simulink model "GCU_Model_genCode"  (R2018a)
settings: Solver=FixedStepDiscrete  StartTime=0.0  StopTime=20  FixedStep=0.0002  RelTol=1e-3  EnableMultiTasking=on
libraries: simulink x3, uartLib x2, clutchMotorLib x1, efiLib x1, engineControlLib x1, gearMotorLib x1
(part 1 of 2)
settings Model: Creator=SIMONE  LastModifiedBy=SIMONE
settings SolverCC: AutoInsertRateTranBlk=on
settings OptimizationCC: DefaultParameterBehavior=Inlined  UseDivisionForNetSlopeComputation=on  UseFloatMulNetSlope=on  InlineInvariantSignals=on  PassReuseOutputArgsAs=Individual arguments  ZeroExternalMemoryAtStartup=off  ZeroInternalMemoryAtStartup=off  NoFixptDivByZeroProtection=on  EfficientFloat2IntCast=on  LifeSpan=1  OptimizeBlockOrder=speed  DifferentSizesBufferReuse=on
settings DebuggingCC: ParameterTunabilityLossMsg=error
settings HardwareCC: ProdBitPerPointer=32  ProdBitPerSizeT=32  ProdBitPerPtrDiffT=32  ProdLargestAtomicInteger=Long  ProdLargestAtomicFloat=Double  ProdWordSize=32  ProdLongLongMode=on  ProdHWDeviceType=ARM Compatible->ARM Cortex
settings SFSimCC: MATLABDynamicMemAlloc=off
settings RTWCC: SystemTargetFile=ert.tlc  TemplateMakefile=ert_default_tmf  GenerateReport=on  IncludeHyperlinkInReport=on  LaunchReport=on  GenerateTraceInfo=on  GenerateTraceReport=on  GenerateTraceReportSl=on  GenerateTraceReportSf=on  GenerateTraceReportEml=on  GenerateCodeMetricsReport=on
settings CodeAppCC: ForceParamTrailComments=on  IgnoreCustomStorageClasses=off  OperatorAnnotations=on  SimulinkDataObjDesc=on  SFDataObjDesc=on  CustomSymbolStrGlobalVar=rt$N$M  CustomSymbolStrType=$N$M  CustomSymbolStrFcn=$N$M$F  CustomSymbolStrMacro=$N$M  InsertBlockDesc=on
settings ERTTargetCC: TargetLangStandard=C99 (ISO)  GenerateSampleERTMain=on  IncludeMdlTerminateFcn=off  CombineSignalStateStructs=on  SupportAbsoluteTime=off  SupportComplex=off  SupportNonInlinedSFcns=on  InlinedParameterPlacement=NonHierarchical  ERTCustomFileTemplate=example_file_process.tlc  ERTFilePackagingFormat=CompactWithDataFile  MemSecPackage=Simulink

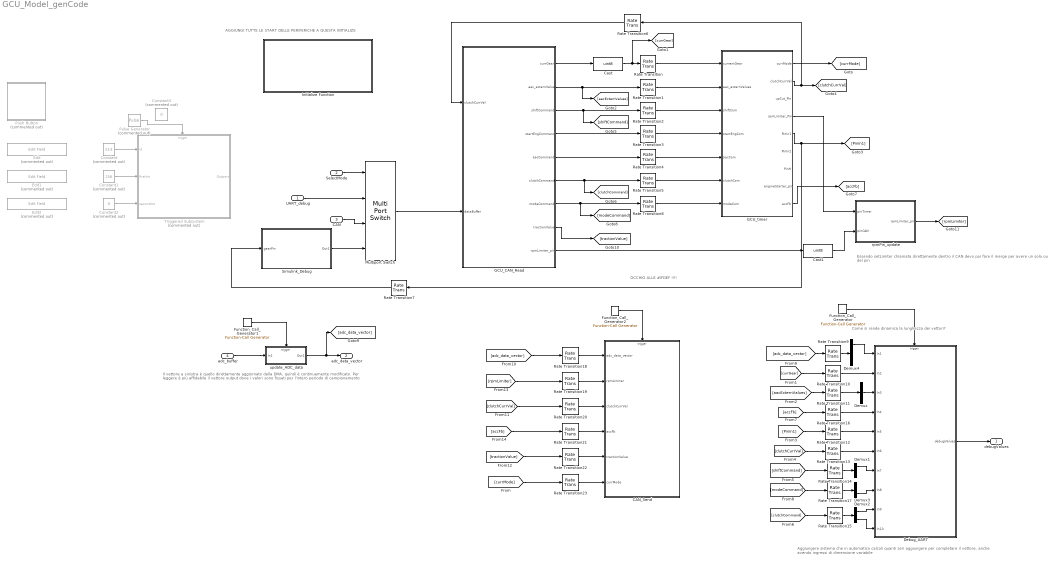
== system GCU_Model_genCode ==
  note: AGGIUNGI TUTTE LE START DELLE PERIFERICHE A QUESTA INITIALIZE
  note: Il vettore a sinistra è quello direttamente aggiornato dalla DMA, quindi è continuamente modificato.
      | Per leggere è più affidabile il vettore output dove i valori sono fissati per l'intero periodo di campionamento
  note: Come si rende dinamica la lunghezza dei vettori?
  note: Essendo setLimiter chiamata direttamente dentro il CAN devo poi fare il merge
      | per avere un solo output del pin
  note: OCCHIO ALLE #IFDEF !!!!
  note: Aggiungere sistema che in automatico calcoli quanti zeri aggiungere
      | per completare il vettore, anche avendo ingressi di dimensione variabile
  UART_debug : Inport  OutDataTypeStr=uint8  PortDimensions=10
  SelectMode : Inport  Port=2
  CAN : Inport  Port=3  OutDataTypeStr=uint8  PortDimensions=10
  adc_buffer : Inport  Port=4  OutDataTypeStr=uint32
  CAN_Send : Subsystem  TreatAsAtomicUnit=on
  Cast : DataTypeConversion  OutDataTypeStr=uint8
  Cast1 : DataTypeConversion  OutDataTypeStr=uint8
  Constant : Constant  Commented=on  Value=513  OutDataTypeStr=uint16
  Constant1 : Constant  Commented=on  Value=256  OutDataTypeStr=uint16
  Constant2 : Constant  Commented=on  Value=0  OutDataTypeStr=uint16
  Constant3 : Constant  Commented=on  Value=0
  "Debug_UART " : Subsystem  TreatAsAtomicUnit=on
  Demux : Demux  Outputs=3
  Demux1 : Demux  Outputs=2
  Demux2 : Demux  Outputs=2
  Demux3 : Demux  Outputs=2
  Demux4 : Demux  Outputs=10
  Edit : EditField  Commented=on  WebBlockId=879  LabelPosition=Hide  Alignment=Center
  Edit1 : EditField  Commented=on  WebBlockId=880  LabelPosition=Hide  Alignment=Center
  Edit2 : EditField  Commented=on  WebBlockId=881  LabelPosition=Hide  Alignment=Center
  Function_Call_Generator : simulink/Ports & Subsystems/Function-Call Generator  sample_time=[0.001, 0.0004]  numberOfIterations=1
  Function_Call_Generator1 : simulink/Ports & Subsystems/Function-Call Generator  sample_time=[0.001, 0.0006]  numberOfIterations=1
  Function_Call_Generator2 : simulink/Ports & Subsystems/Function-Call Generator  sample_time=[0.001, 0.0008]  numberOfIterations=1
  GCU_CAN_Read : Subsystem  TreatAsAtomicUnit=on  SystemSampleTime=[0.001, 0.0002]
  GCU_timer : Subsystem  TreatAsAtomicUnit=on  SystemSampleTime=0.001
  Initialize Function : Subsystem  TreatAsAtomicUnit=on
  Multiport Switch : MultiPortSwitch  DiagnosticForDefault=Warning
  Pulse Generator : DiscretePulseGenerator  Commented=on  PulseType=Time based  Period=1000  PulseWidth=0.1  PhaseDelay=1
  Push Button : Subsystem  Commented=on  DialogController=hmiCreateDDGDialog  IsWebBlock=on  mask(MWDashboardBlock){webBlockId=12b47424-de0c-4dac-be92-db9266863398, webBlockType=pushbutton, ShowInLibBrwoser=on, ShowInitialText=on, HMISrcModelName=GCU_Model_genCode}
      mask prompts: webBlockId "WebBlock Id"; webBlockType "WebBlock Type"; HMISrcModelName "Source Model"
      mask help: SimulinkHMI:dialogs:PushButtonDialogDesc
      mask Help: helpview([docroot '/mapfiles/simulink.map'], 'hmi_push_button')
      mask Display:
      | model = bdroot(gcb);
      | if strcmp(get_param(model,'BlockDiagramType'), 'library')
      |     image([(matlabroot) '/toolbox/simulink/hmi/icons/PushButton.png']);
      | end
  Rate Transition{,1..23} (24 alike) : RateTransition  Deterministic=off
  Simulink_Debug : Subsystem  TreatAsAtomicUnit=on  SystemSampleTime=[0.001, 0.0002]
  Triggered Subsystem : Subsystem  Commented=on  TreatAsAtomicUnit=on
  rpmPin_update : Subsystem
  update_ADC_data : Subsystem  TreatAsAtomicUnit=on
  "debugValues " : Outport
  adc_data_vector : Outport  Port=2  OutDataTypeStr=uint32
  wires:
  GCU_CAN_Read/9(rpmLimiter_pin) -> Cast1/1
  GCU_CAN_Read/4(startEngCommand) -> Rate Transition3/1
  Multiport Switch/1 -> GCU_CAN_Read/2(dataBuffer)
  Rate Transition8/1 -> GCU_timer/7(modeCom)
  Rate Transition/1 -> GCU_timer/1(currentGear)
  Cast/1 -> [currGear], Rate Transition/1
  GCU_CAN_Read/7(modeCommand) -> [modeCommand], Rate Transition8/1
  GCU_timer/5(PinIn1) -> Rate Transition7/1, [PinIn1]
  Rate Transition4/1 -> GCU_timer/5(aacCom)
  GCU_CAN_Read/2(aac_externValue) -> [aacExternValues], Rate Transition1/1
  GCU_CAN_Read/3(shiftCommand) -> [shiftCommand], Rate Transition2/1
  GCU_timer/2(clutchCurrVal) -> [clutchCurrVal], Rate Transition6/1
  Cast1/1 -> rpmPin_update/2(pinCAN)
  Rate Transition5/1 -> GCU_timer/6(clutchCom)
  GCU_CAN_Read/1(currGear) -> Cast/1
  Rate Transition2/1 -> GCU_timer/3(shiftCom)
  Rate Transition1/1 -> GCU_timer/2(aac_externValues)
  GCU_timer/4(rpmLimiter_Pin) -> rpmPin_update/1(pinTimer)
  GCU_CAN_Read/6(clutchCommand) -> [clutchCommand], Rate Transition5/1
  GCU_CAN_Read/5(aacCommand) -> Rate Transition4/1
  Rate Transition6/1 -> GCU_CAN_Read/1(clutchCurrVal)
  Rate Transition3/1 -> GCU_timer/4(startEngCom)
  Function_Call_Generator/1 -> "Debug_UART "/Trigger
  "Debug_UART "/1(debugValues) -> "debugValues "/1
  Rate Transition10/1 -> "Debug_UART "/2(In2)
  Rate Transition11/1 -> Demux/1
  Demux/2 -> "Debug_UART "/3(In3)
  Rate Transition7/1 -> Simulink_Debug/1(gearPin)
  Simulink_Debug/1(Out1) -> Multiport Switch/4
  GCU_timer/1(currMode) -> [currMode]
  [currGear] -> Rate Transition10/1
  [aacExternValues] -> Rate Transition11/1
  [PinIn1] -> Rate Transition12/1
  Rate Transition12/1 -> "Debug_UART "/5(In5)
  [clutchCurrVal] -> Rate Transition13/1
  Rate Transition13/1 -> "Debug_UART "/6(In6)
  [shiftCommand] -> Rate Transition14/1
  [clutchCommand] -> Rate Transition15/1
  Rate Transition14/1 -> Demux1/1
  Demux1/1 -> "Debug_UART "/7(In7)
  Demux2/1 -> "Debug_UART "/9(In9)
  Rate Transition15/1 -> Demux2/1
  Demux2/2 -> "Debug_UART "/10(In10)
  Constant/1 -> Triggered Subsystem/1(id)
  Constant2/1 -> Triggered Subsystem/3(secondInt)
  Constant1/1 -> Triggered Subsystem/2(firstInt)
  Pulse Generator/1 -> Triggered Subsystem/Trigger
  SelectMode/1 -> Multiport Switch/1
  UART_debug/1 -> Multiport Switch/2
  GCU_timer/9(accFb) -> [accFb]
  [accFb] -> Rate Transition16/1
  Rate Transition16/1 -> "Debug_UART "/4(In4)
  [modeCommand] -> Rate Transition17/1
  Rate Transition17/1 -> Demux3/1
  Demux3/2 -> "Debug_UART "/8(In8)
  CAN/1 -> Multiport Switch/3
  Function_Call_Generator1/1 -> update_ADC_data/Trigger
  adc_buffer/1 -> update_ADC_data/1(In1)
  update_ADC_data/1(Out1) -> [adc_data_vector], adc_data_vector/1
  [adc_data_vector] -> Rate Transition9/1
  Rate Transition9/1 -> Demux4/1
  Demux4/1 -> "Debug_UART "/1(In1)
  Function_Call_Generator2/1 -> CAN_Send/Trigger
  [adc_data_vector] -> Rate Transition18/1
  GCU_CAN_Read/8(tractionValue) -> [tractionValue]
  [currMode] -> Rate Transition23/1
  [clutchCurrVal] -> Rate Transition20/1
  [tractionValue] -> Rate Transition22/1
  rpmPin_update/1(rpmLimiter_pin) -> [rpmLimiter]
  [rpmLimiter] -> Rate Transition19/1
  [accFb] -> Rate Transition21/1
  Rate Transition18/1 -> CAN_Send/1(adc_data_vector)
  Rate Transition19/1 -> CAN_Send/2(rpmLimiter)
  Rate Transition20/1 -> CAN_Send/3(clutchCurrVal)
  Rate Transition21/1 -> CAN_Send/4(accFb)
  Rate Transition22/1 -> CAN_Send/5(tractionValue)
  Rate Transition23/1 -> CAN_Send/6(currMode)

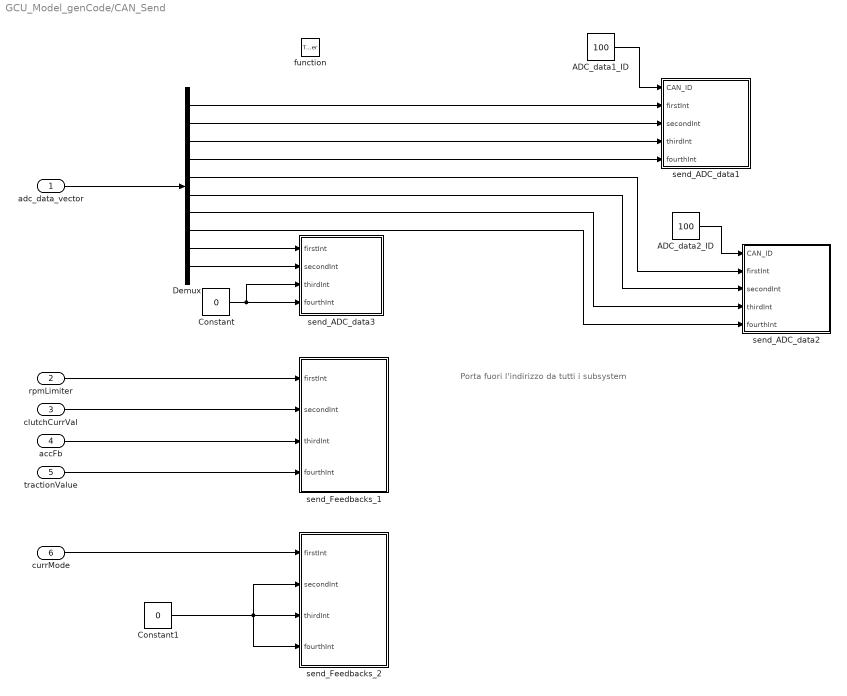
== system GCU_Model_genCode/CAN_Send ==
  note: Porta fuori l'indirizzo da tutti i subsystem
  adc_data_vector : Inport
  rpmLimiter : Inport  Port=2
  clutchCurrVal : Inport  Port=3
  accFb : Inport  Port=4
  tractionValue : Inport  Port=5
  currMode : Inport  Port=6
  function : TriggerPort  TriggerType=function-call  VariantControl=Variant
  ADC_data1_ID : Constant  Value=100  OutDataTypeStr=uint16
  ADC_data2_ID : Constant  Value=100  OutDataTypeStr=uint16
  Constant : Constant  Value=0  OutDataTypeStr=uint16
  Constant1 : Constant  Value=0  OutDataTypeStr=uint16
  Demux : Demux  Outputs=10
  send_ADC_data1 : Subsystem
  send_ADC_data2 : Subsystem
  send_ADC_data3 : Subsystem
  send_Feedbacks_1 : Subsystem
  send_Feedbacks_2 : Subsystem
  wires:
  adc_data_vector/1 -> Demux/1
  Demux/1 -> send_ADC_data1/2(firstInt)
  Demux/2 -> send_ADC_data1/3(secondInt)
  Demux/3 -> send_ADC_data1/4(thirdInt)
  Demux/4 -> send_ADC_data1/5(fourthInt)
  Demux/5 -> send_ADC_data2/2(firstInt)
  Demux/6 -> send_ADC_data2/3(secondInt)
  Demux/7 -> send_ADC_data2/4(thirdInt)
  Demux/8 -> send_ADC_data2/5(fourthInt)
  Demux/9 -> send_ADC_data3/1(firstInt)
  Demux/10 -> send_ADC_data3/2(secondInt)
  Constant/1 -> send_ADC_data3/3(thirdInt), send_ADC_data3/4(fourthInt)
  rpmLimiter/1 -> send_Feedbacks_1/1(firstInt)
  clutchCurrVal/1 -> send_Feedbacks_1/2(secondInt)
  accFb/1 -> send_Feedbacks_1/3(thirdInt)
  tractionValue/1 -> send_Feedbacks_1/4(fourthInt)
  currMode/1 -> send_Feedbacks_2/1(firstInt)
  Constant1/1 -> send_Feedbacks_2/4(fourthInt), send_Feedbacks_2/2(secondInt), send_Feedbacks_2/3(thirdInt)
  ADC_data1_ID/1 -> send_ADC_data1/1(CAN_ID)
  ADC_data2_ID/1 -> send_ADC_data2/1(CAN_ID)

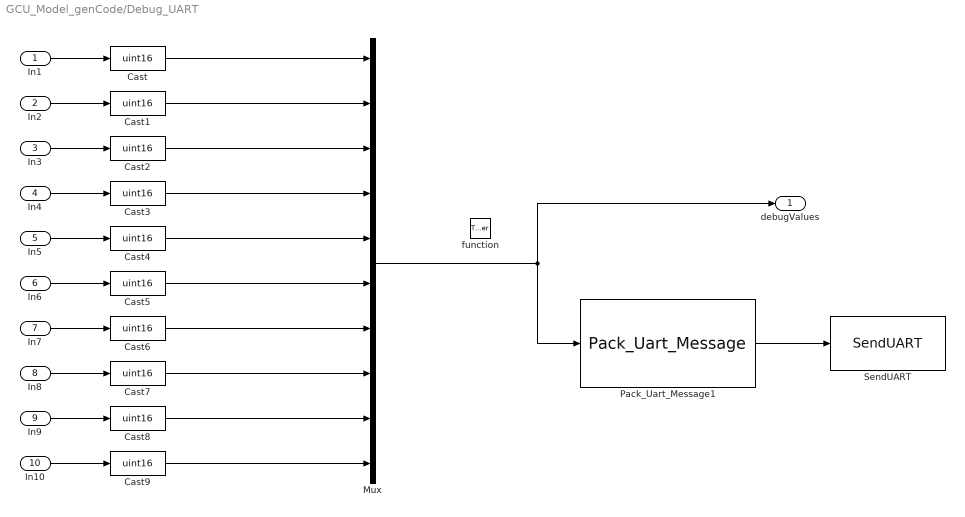
== system GCU_Model_genCode/Debug_UART  ==
  In1 : Inport
  In2 : Inport  Port=2
  In3 : Inport  Port=3
  In4 : Inport  Port=4
  In5 : Inport  Port=5
  In6 : Inport  Port=6
  In7 : Inport  Port=7
  In8 : Inport  Port=8
  In9 : Inport  Port=9
  In10 : Inport  Port=10
  function : TriggerPort  TriggerType=function-call  VariantControl=Variant
  Cast{,1..9} (10 alike) : DataTypeConversion  OutDataTypeStr=uint16
  Mux : Mux  Inputs=10
  Pack_Uart_Message1 : uartLib/Pack_Uart_Message  SFunctionModules=''
      settings: SourceProductName=GCU Library
  SendUART : uartLib/SendUART  SFunctionModules=''
      settings: SourceProductName=GCU Library
  debugValues : Outport
  wires:
  Pack_Uart_Message1/1 -> SendUART/1
  Mux/1 -> debugValues/1, Pack_Uart_Message1/1
  In1/1 -> Cast/1
  Cast/1 -> Mux/1
  In2/1 -> Cast1/1
  Cast1/1 -> Mux/2
  In3/1 -> Cast2/1
  Cast2/1 -> Mux/3
  Cast3/1 -> Mux/4
  In4/1 -> Cast3/1
  Cast4/1 -> Mux/5
  In5/1 -> Cast4/1
  Cast5/1 -> Mux/6
  In6/1 -> Cast5/1
  Cast6/1 -> Mux/7
  In7/1 -> Cast6/1
  Cast7/1 -> Mux/8
  In8/1 -> Cast7/1
  Cast8/1 -> Mux/9
  In9/1 -> Cast8/1
  Cast9/1 -> Mux/10
  In10/1 -> Cast9/1

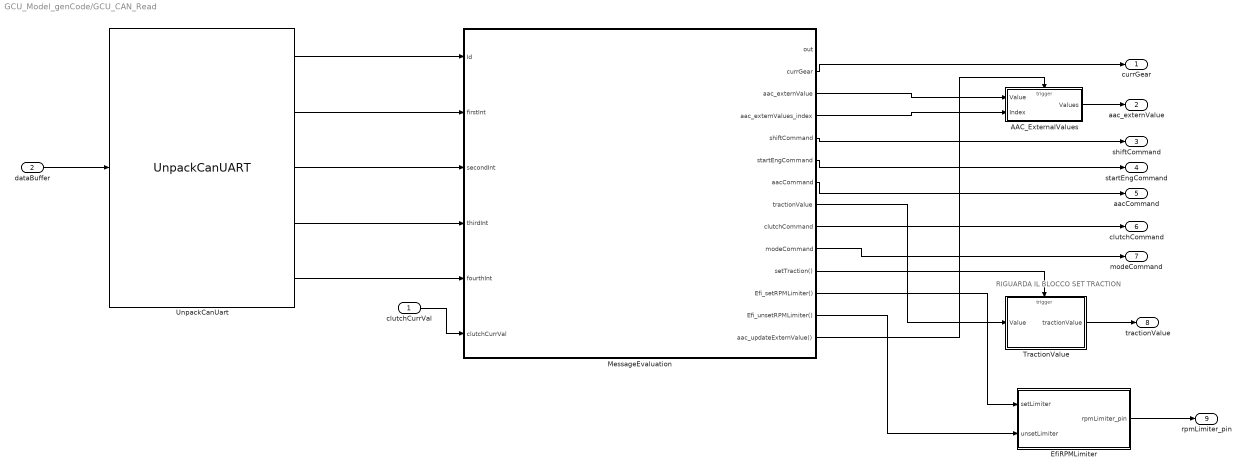
== system GCU_Model_genCode/GCU_CAN_Read ==
  note: RIGUARDA IL BLOCCO SET TRACTION
  clutchCurrVal : Inport
  dataBuffer : Inport  Port=2
  AAC_ExternalValues : Subsystem  TreatAsAtomicUnit=on
  EfiRPMLimiter : Subsystem
  MessageEvaluation : Stateflow chart  TreatAsAtomicUnit=on  SystemSampleTime=[0.001, 0.0002]
  TractionValue : Subsystem  TreatAsAtomicUnit=on
  UnpackCanUart : S-Function  FunctionName=UnpackCanUART  SFunctionDeploymentMode=off  EnableBusSupport=off
  currGear : Outport
  aac_externValue : Outport  Port=2
  shiftCommand : Outport  Port=3
  startEngCommand : Outport  Port=4
  aacCommand : Outport  Port=5
  clutchCommand : Outport  Port=6
  modeCommand : Outport  Port=7
  tractionValue : Outport  Port=8
  rpmLimiter_pin : Outport  Port=9
  wires:
  MessageEvaluation/12(Efi_setRPMLimiter()) -> EfiRPMLimiter/1(setLimiter)
  UnpackCanUart/4 -> MessageEvaluation/4(thirdInt)
  MessageEvaluation/4(aac_externValues_index) -> AAC_ExternalValues/2(Index)
  MessageEvaluation/13(Efi_unsetRPMLimiter()) -> EfiRPMLimiter/2(unsetLimiter)
  MessageEvaluation/7(aacCommand) -> aacCommand/1
  MessageEvaluation/9(clutchCommand) -> clutchCommand/1
  dataBuffer/1 -> UnpackCanUart/1
  MessageEvaluation/10(modeCommand) -> modeCommand/1
  MessageEvaluation/11(setTraction()) -> TractionValue/Trigger
  MessageEvaluation/5(shiftCommand) -> shiftCommand/1
  MessageEvaluation/3(aac_externValue) -> AAC_ExternalValues/1(Value)
  MessageEvaluation/8(tractionValue) -> TractionValue/1(Value)
  MessageEvaluation/6(startEngCommand) -> startEngCommand/1
  UnpackCanUart/1 -> MessageEvaluation/1(Id)
  UnpackCanUart/5 -> MessageEvaluation/5(fourthInt)
  TractionValue/1(tractionValue) -> tractionValue/1
  UnpackCanUart/3 -> MessageEvaluation/3(secondInt)
  clutchCurrVal/1 -> MessageEvaluation/6(clutchCurrVal)
  MessageEvaluation/2(currGear) -> currGear/1
  MessageEvaluation/14(aac_updateExternValue()) -> AAC_ExternalValues/Trigger
  UnpackCanUart/2 -> MessageEvaluation/2(firstInt)
  EfiRPMLimiter/1(rpmLimiter_pin) -> rpmLimiter_pin/1
  AAC_ExternalValues/1(Values) -> aac_externValue/1

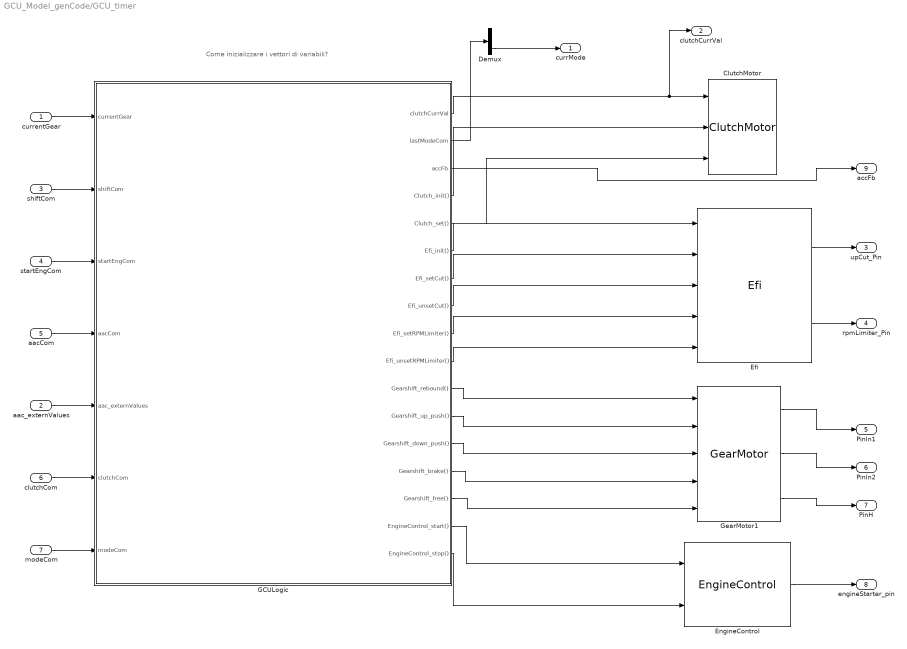
== system GCU_Model_genCode/GCU_timer ==
  note: Come inizializzare i vettori di variabili?
  currentGear : Inport
  aac_externValues : Inport  Port=2
  shiftCom : Inport  Port=3
  startEngCom : Inport  Port=4
  aacCom : Inport  Port=5
  clutchCom : Inport  Port=6
  modeCom : Inport  Port=7
  ClutchMotor : clutchMotorLib/ClutchMotor  SystemSampleTime=-1
      settings: SourceProductName=GCU Library
  Demux : Demux  Outputs=2
  Efi : efiLib/Efi
      settings: SourceProductName=GCU Library
  EngineControl : engineControlLib/EngineControl
      settings: SourceProductName=GCU Library
  GCULogic : Stateflow chart  TreatAsAtomicUnit=on
  GearMotor1 : gearMotorLib/GearMotor
      settings: SourceProductName=GCU Library
  currMode : Outport
  clutchCurrVal : Outport  Port=2
  upCut_Pin : Outport  Port=3
  rpmLimiter_Pin : Outport  Port=4
  PinIn1 : Outport  Port=5
  PinIn2 : Outport  Port=6
  PinH : Outport  Port=7
  engineStarter_pin : Outport  Port=8
  accFb : Outport  Port=9
  wires:
  GCULogic/17(EngineControl_stop()) -> EngineControl/2
  startEngCom/1 -> GCULogic/3(startEngCom)
  GCULogic/9(Efi_setRPMLimiter()) -> Efi/4
  GCULogic/6(Efi_init()) -> Efi/1
  clutchCom/1 -> GCULogic/6(clutchCom)
  GCULogic/16(EngineControl_start()) -> EngineControl/1
  GearMotor1/3 -> PinH/1
  GCULogic/10(Efi_unsetRPMLimiter()) -> Efi/5
  EngineControl/1 -> engineStarter_pin/1
  GCULogic/15(Gearshift_free()) -> GearMotor1/5
  GCULogic/14(Gearshift_brake()) -> GearMotor1/4
  GCULogic/11(Gearshift_rebound()) -> GearMotor1/1
  GearMotor1/2 -> PinIn2/1
  GearMotor1/1 -> PinIn1/1
  GCULogic/12(Gearshift_up_push()) -> GearMotor1/2
  shiftCom/1 -> GCULogic/2(shiftCom)
  aacCom/1 -> GCULogic/4(aacCom)
  GCULogic/4(Clutch_init()) -> ClutchMotor/2
  Efi/2 -> rpmLimiter_Pin/1
  GCULogic/7(Efi_setCut()) -> Efi/2
  Efi/1 -> upCut_Pin/1
  currentGear/1 -> GCULogic/1(currentGear)
  GCULogic/1(clutchCurrVal) -> ClutchMotor/1, clutchCurrVal/1
  GCULogic/8(Efi_unsetCut()) -> Efi/3
  GCULogic/5(Clutch_set()) -> ClutchMotor/3
  modeCom/1 -> GCULogic/7(modeCom)
  aac_externValues/1 -> GCULogic/5(aac_externValues)
  GCULogic/13(Gearshift_down_push()) -> GearMotor1/3
  GCULogic/3(accFb) -> accFb/1
  GCULogic/2(lastModeCom) -> Demux/1
  Demux/2 -> currMode/1

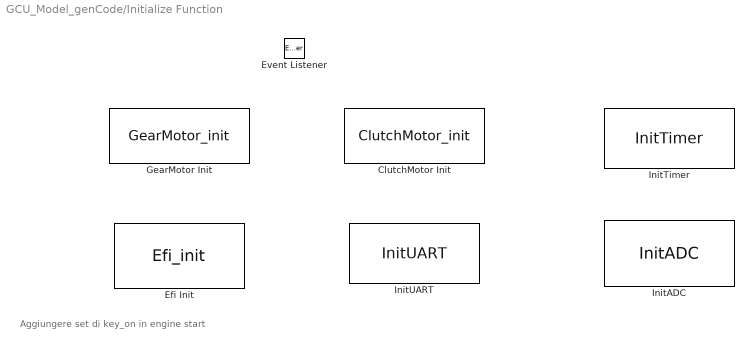
== system GCU_Model_genCode/Initialize Function ==
  note: Aggiungere set di key_on in engine start
  ClutchMotor Init : S-Function  FunctionName=ClutchMotor_init  SFunctionDeploymentMode=off  EnableBusSupport=off
  Efi Init : S-Function  FunctionName=Efi_init  SFunctionDeploymentMode=off  EnableBusSupport=off
  Event Listener : EventListener  DisableCoverage=on  EventName=reset
  GearMotor Init : S-Function  FunctionName=GearMotor_init  SFunctionDeploymentMode=off  EnableBusSupport=off
  InitADC : S-Function  FunctionName=InitADC  SFunctionDeploymentMode=off  EnableBusSupport=off
  InitTimer : S-Function  FunctionName=InitTimer  SFunctionDeploymentMode=off  EnableBusSupport=off
  InitUART : S-Function  FunctionName=InitUART  SFunctionDeploymentMode=off  EnableBusSupport=off

== system GCU_Model_genCode/Push Button ==

== system GCU_Model_genCode/Simulink_Debug ==
  gearPin : Inport
  AccelerationRoutine : Stateflow chart  TreatAsAtomicUnit=on  SystemSampleTime=[0.001, 0.0002]
  PackCanUart : S-Function  FunctionName=PackCanUART  SFunctionDeploymentMode=off  EnableBusSupport=off
  Out1 : Outport
  wires:
  PackCanUart/1 -> Out1/1
  AccelerationRoutine/2(firstInt) -> PackCanUart/2
  AccelerationRoutine/1(id) -> PackCanUart/1
  AccelerationRoutine/3(secondInt) -> PackCanUart/3
  gearPin/1 -> AccelerationRoutine/1(gearPin)

== system GCU_Model_genCode/Triggered Subsystem ==
  id : Inport
  firstInt : Inport  Port=2
  secondInt : Inport  Port=3
  Trigger : TriggerPort  VariantControl=Variant
  PackCanUart : S-Function  FunctionName=PackCanUART  SFunctionDeploymentMode=off  EnableBusSupport=off
  Scope : Scope
  Outport : Outport
  wires:
  PackCanUart/1 -> Outport/1, Scope/1
  id/1 -> PackCanUart/1
  firstInt/1 -> PackCanUart/2
  secondInt/1 -> PackCanUart/3

== system GCU_Model_genCode/rpmPin_update ==
  pinTimer : Inport
  pinCAN : Inport  Port=2
  Merge : Merge
  Rate Transition : RateTransition  Deterministic=off
  Triggered_Subsystem : Subsystem  TreatAsAtomicUnit=on
  Triggered_Subsystem1 : Subsystem  TreatAsAtomicUnit=on
  rpmLimiter_pin : Outport
  wires:
  pinTimer/1 -> Triggered_Subsystem/1(In1), Triggered_Subsystem/Trigger
  pinCAN/1 -> Rate Transition/1
  Triggered_Subsystem/1(Out1) -> Merge/1
  Triggered_Subsystem1/1(Out1) -> Merge/2
  Merge/1 -> rpmLimiter_pin/1
  Rate Transition/1 -> Triggered_Subsystem1/1(In1), Triggered_Subsystem1/Trigger

== system GCU_Model_genCode/update_ADC_data ==
  In1 : Inport
  function : TriggerPort  TriggerType=function-call  VariantControl=Variant
  update_ADC_data : S-Function  FunctionName=update_ADC_data  SFunctionDeploymentMode=off  EnableBusSupport=off
  Out1 : Outport
  wires:
  In1/1 -> update_ADC_data/1
  update_ADC_data/1 -> Out1/1

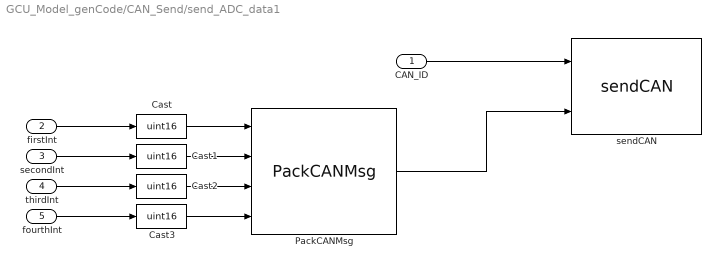
== system GCU_Model_genCode/CAN_Send/send_ADC_data1 ==
  CAN_ID : Inport
  firstInt : Inport  Port=2
  secondInt : Inport  Port=3
  thirdInt : Inport  Port=4
  fourthInt : Inport  Port=5
  Cast{,1..3} (4 alike) : DataTypeConversion  OutDataTypeStr=uint16
  PackCANMsg : S-Function  FunctionName=PackCANMsg  SFunctionDeploymentMode=off  EnableBusSupport=off
  sendCAN : S-Function  FunctionName=sendCAN  SFunctionDeploymentMode=off  EnableBusSupport=off
  wires:
  CAN_ID/1 -> sendCAN/1
  PackCANMsg/1 -> sendCAN/2
  firstInt/1 -> Cast/1
  secondInt/1 -> Cast1/1
  thirdInt/1 -> Cast2/1
  fourthInt/1 -> Cast3/1
  Cast/1 -> PackCANMsg/1
  Cast1/1 -> PackCANMsg/2
  Cast2/1 -> PackCANMsg/3
  Cast3/1 -> PackCANMsg/4

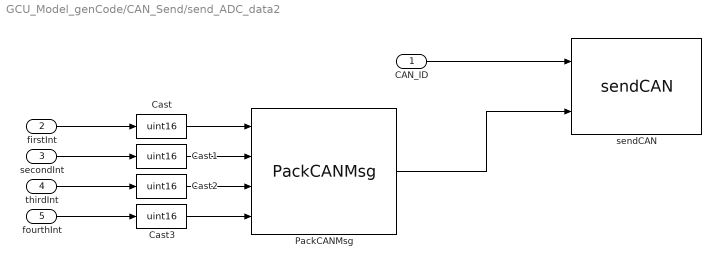
== system GCU_Model_genCode/CAN_Send/send_ADC_data2 ==
  CAN_ID : Inport
  firstInt : Inport  Port=2
  secondInt : Inport  Port=3
  thirdInt : Inport  Port=4
  fourthInt : Inport  Port=5
  Cast{,1..3} (4 alike) : DataTypeConversion  OutDataTypeStr=uint16
  PackCANMsg : S-Function  FunctionName=PackCANMsg  SFunctionDeploymentMode=off  EnableBusSupport=off
  sendCAN : S-Function  FunctionName=sendCAN  SFunctionDeploymentMode=off  EnableBusSupport=off
  wires:
  CAN_ID/1 -> sendCAN/1
  PackCANMsg/1 -> sendCAN/2
  firstInt/1 -> Cast/1
  secondInt/1 -> Cast1/1
  thirdInt/1 -> Cast2/1
  fourthInt/1 -> Cast3/1
  Cast/1 -> PackCANMsg/1
  Cast1/1 -> PackCANMsg/2
  Cast2/1 -> PackCANMsg/3
  Cast3/1 -> PackCANMsg/4

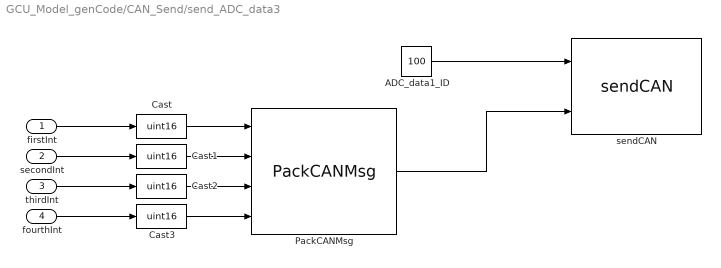
== system GCU_Model_genCode/CAN_Send/send_ADC_data3 ==
  firstInt : Inport
  secondInt : Inport  Port=2
  thirdInt : Inport  Port=3
  fourthInt : Inport  Port=4
  ADC_data1_ID : Constant  Value=100  OutDataTypeStr=uint16
  Cast{,1..3} (4 alike) : DataTypeConversion  OutDataTypeStr=uint16
  PackCANMsg : S-Function  FunctionName=PackCANMsg  SFunctionDeploymentMode=off  EnableBusSupport=off
  sendCAN : S-Function  FunctionName=sendCAN  SFunctionDeploymentMode=off  EnableBusSupport=off
  wires:
  ADC_data1_ID/1 -> sendCAN/1
  PackCANMsg/1 -> sendCAN/2
  firstInt/1 -> Cast/1
  secondInt/1 -> Cast1/1
  thirdInt/1 -> Cast2/1
  fourthInt/1 -> Cast3/1
  Cast/1 -> PackCANMsg/1
  Cast1/1 -> PackCANMsg/2
  Cast2/1 -> PackCANMsg/3
  Cast3/1 -> PackCANMsg/4

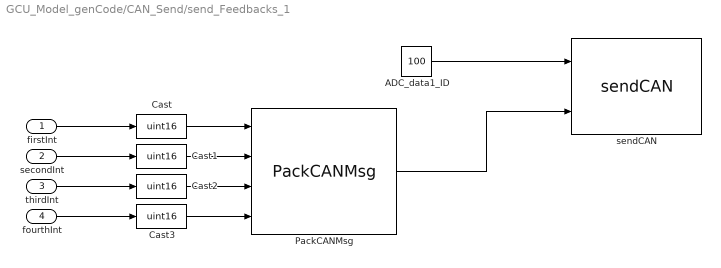
== system GCU_Model_genCode/CAN_Send/send_Feedbacks_1 ==
  firstInt : Inport
  secondInt : Inport  Port=2
  thirdInt : Inport  Port=3
  fourthInt : Inport  Port=4
  ADC_data1_ID : Constant  Value=100  OutDataTypeStr=uint16
  Cast{,1..3} (4 alike) : DataTypeConversion  OutDataTypeStr=uint16
  PackCANMsg : S-Function  FunctionName=PackCANMsg  SFunctionDeploymentMode=off  EnableBusSupport=off
  sendCAN : S-Function  FunctionName=sendCAN  SFunctionDeploymentMode=off  EnableBusSupport=off
  wires:
  ADC_data1_ID/1 -> sendCAN/1
  PackCANMsg/1 -> sendCAN/2
  firstInt/1 -> Cast/1
  secondInt/1 -> Cast1/1
  thirdInt/1 -> Cast2/1
  fourthInt/1 -> Cast3/1
  Cast/1 -> PackCANMsg/1
  Cast1/1 -> PackCANMsg/2
  Cast2/1 -> PackCANMsg/3
  Cast3/1 -> PackCANMsg/4

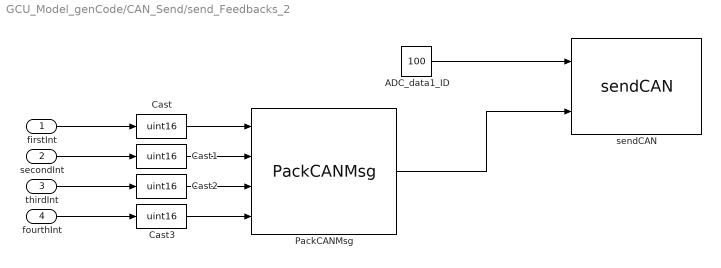
== system GCU_Model_genCode/CAN_Send/send_Feedbacks_2 ==
  firstInt : Inport
  secondInt : Inport  Port=2
  thirdInt : Inport  Port=3
  fourthInt : Inport  Port=4
  ADC_data1_ID : Constant  Value=100  OutDataTypeStr=uint16
  Cast{,1..3} (4 alike) : DataTypeConversion  OutDataTypeStr=uint16
  PackCANMsg : S-Function  FunctionName=PackCANMsg  SFunctionDeploymentMode=off  EnableBusSupport=off
  sendCAN : S-Function  FunctionName=sendCAN  SFunctionDeploymentMode=off  EnableBusSupport=off
  wires:
  ADC_data1_ID/1 -> sendCAN/1
  PackCANMsg/1 -> sendCAN/2
  firstInt/1 -> Cast/1
  secondInt/1 -> Cast1/1
  thirdInt/1 -> Cast2/1
  fourthInt/1 -> Cast3/1
  Cast/1 -> PackCANMsg/1
  Cast1/1 -> PackCANMsg/2
  Cast2/1 -> PackCANMsg/3
  Cast3/1 -> PackCANMsg/4

== system GCU_Model_genCode/GCU_CAN_Read/AAC_ExternalValues ==
  Value : Inport
  Index : Inport  Port=2
  function : TriggerPort  TriggerType=function-call  VariantControl=Variant
  Assignment : Assignment  IndexMode=Zero-based  DiagnosticForDimensions=Warning  IndexOptions=Index vector (port)  Indices=1  OutputSizes=1
  Unit Delay : UnitDelay  InitialCondition=[0,0,0]  SampleTime=-1
  Values : Outport
  wires:
  Assignment/1 -> Unit Delay/1, Values/1
  Unit Delay/1 -> Assignment/1
  Value/1 -> Assignment/2
  Index/1 -> Assignment/3

== system GCU_Model_genCode/GCU_CAN_Read/EfiRPMLimiter ==
  setLimiter : Inport
  unsetLimiter : Inport  Port=2
  Efi_setRpmLimiter : Subsystem  TreatAsAtomicUnit=on
  Efi_unsetRpmLimiter : Subsystem  TreatAsAtomicUnit=on
  Merge : Merge
  rpmLimiter_pin : Outport
  wires:
  setLimiter/1 -> Efi_setRpmLimiter/Trigger
  unsetLimiter/1 -> Efi_unsetRpmLimiter/Trigger
  Efi_unsetRpmLimiter/1(rpmLimiter_pin) -> Merge/2
  Efi_setRpmLimiter/1(rpmLimiter_pin) -> Merge/1
  Merge/1 -> rpmLimiter_pin/1

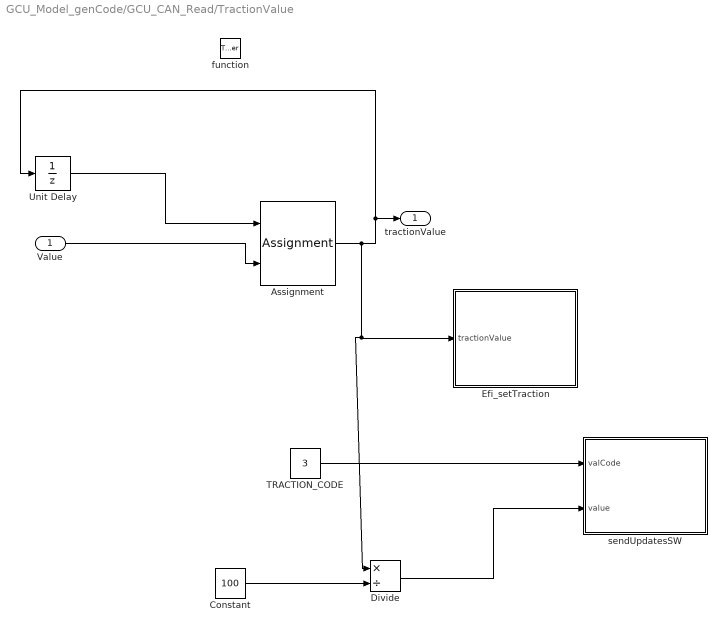
== system GCU_Model_genCode/GCU_CAN_Read/TractionValue ==
  Value : Inport
  function : TriggerPort  TriggerType=function-call  VariantControl=Variant
  Assignment : Assignment  IndexMode=Zero-based  DiagnosticForDimensions=Warning  IndexOptions=Index vector (dialog)  Indices=0  OutputSizes=1
  Constant : Constant  Value=100  OutDataTypeStr=uint16
  Divide : Product  Inputs=*/
  Efi_setTraction : Subsystem
  TRACTION_CODE : Constant  Value=3  OutDataTypeStr=uint16
  Unit Delay : UnitDelay  SampleTime=-1
  sendUpdatesSW : Subsystem
  tractionValue : Outport
  wires:
  Value/1 -> Assignment/2
  Assignment/1 -> Divide/1, Efi_setTraction/1(tractionValue), Unit Delay/1, tractionValue/1
  Unit Delay/1 -> Assignment/1
  TRACTION_CODE/1 -> sendUpdatesSW/1(valCode)
  Constant/1 -> Divide/2
  Divide/1 -> sendUpdatesSW/2(value)

== system GCU_Model_genCode/GCU_timer/GCULogic/sendUpdatesSW ==
  valCode : Inport  OutDataTypeStr=uint16  PortDimensions=1
  value : Inport  Port=2  OutDataTypeStr=uint16  PortDimensions=1
  f : TriggerPort  TriggerType=function-call  VariantControl=(inherit)
      settings: CopyFcn=Stateflow.SLINSF.SimulinkMan.removeBlockPreDeleteFcn  PreDeleteFcn=Stateflow.SLINSF.SimulinkMan.unsafePredeleteFcn
  GCU_FEEDBACK_ID : Constant  Value=793  OutDataTypeStr=uint16
  PackCanUart : S-Function  FunctionName=PackCanUART  SFunctionDeploymentMode=off  EnableBusSupport=off
  wires:
  GCU_FEEDBACK_ID/1 -> PackCanUart/1
  valCode/1 -> PackCanUart/2
  value/1 -> PackCanUart/3

== system GCU_Model_genCode/rpmPin_update/Triggered_Subsystem ==
  In1 : Inport
  Trigger : TriggerPort  TriggerType=either  VariantControl=Variant
  Out1 : Outport
  wires:
  In1/1 -> Out1/1

== system GCU_Model_genCode/rpmPin_update/Triggered_Subsystem1 ==
  In1 : Inport
  Trigger : TriggerPort  TriggerType=either  VariantControl=Variant
  Out1 : Outport
  wires:
  In1/1 -> Out1/1

== system GCU_Model_genCode/GCU_CAN_Read/EfiRPMLimiter/Efi_setRpmLimiter ==
  function : TriggerPort  TriggerType=function-call  VariantControl=Variant
  Efi SetRPMLimiter : S-Function  FunctionName=Efi_setRPMLimiter  SFunctionDeploymentMode=off  EnableBusSupport=off
  rpmLimiter_pin : Outport
  wires:
  Efi SetRPMLimiter/1 -> rpmLimiter_pin/1

== system GCU_Model_genCode/GCU_CAN_Read/EfiRPMLimiter/Efi_unsetRpmLimiter ==
  function : TriggerPort  TriggerType=function-call  VariantControl=Variant
  Efi UnSetRPMLimiter : S-Function  FunctionName=Efi_unsetRPMLimiter  SFunctionDeploymentMode=off  EnableBusSupport=off
  rpmLimiter_pin : Outport
  wires:
  Efi UnSetRPMLimiter/1 -> rpmLimiter_pin/1

== system GCU_Model_genCode/GCU_CAN_Read/TractionValue/Efi_setTraction ==
  tractionValue : Inport  OutDataTypeStr=uint16  PortDimensions=1
  GCU_TRACTION_CONTROL_EFI_ID : Constant  Value=1280  OutDataTypeStr=uint16
  PackCanUart : S-Function  FunctionName=PackCanUART  SFunctionDeploymentMode=off  EnableBusSupport=off
  wires:
  GCU_TRACTION_CONTROL_EFI_ID/1 -> PackCanUart/1
  tractionValue/1 -> PackCanUart/2

== system GCU_Model_genCode/GCU_CAN_Read/TractionValue/sendUpdatesSW ==
  valCode : Inport  OutDataTypeStr=uint16  PortDimensions=1
  value : Inport  Port=2  OutDataTypeStr=uint16  PortDimensions=1
  GCU_FEEDBACK_ID : Constant  Value=793  OutDataTypeStr=uint16
  PackCanUart : S-Function  FunctionName=PackCanUART  SFunctionDeploymentMode=off  EnableBusSupport=off
  wires:
  GCU_FEEDBACK_ID/1 -> PackCanUart/1
  value/1 -> PackCanUart/3
  valCode/1 -> PackCanUart/2

== stateflow chart GCU_Model_genCode/GCU_timer/GCULogic ==
  settings: updateMethod=DISCRETE  sampleTime=0.001
  state MODES [parallel]
    settings: executionOrder=1
    state MANUAL_MODES
      entry:
      lastModeCom[0] = modeCom[0];
      lastModeCom[1] = modeCom[1];
      entry, during:
      checkShift();
      checkClutch();
      state AUTOCROSS
      state ENDURANCE
      state SKIDPAD
      (default) -> ENDURANCE
    state INIT
    note: numeri delle modalità da decidere
    state checkClutch [function]
      (default) -> (junction 649)
      (junction 649) -> (junction 648) [order 1] : [clutchCom[0] ~= lastClutchCom]
      (junction 649) -> (junction 683) [order 2]
      (junction 648) -> (junction 682)
      (junction 682) -> (junction 687) [order 1] : [(~in(GEARSHIFT.DOWNSHIFTING) && ~in(NEUTRAL_STATE.SET_NEUTRAL)) || in(NEUTRAL_STATE.UNSET_NEUTRAL)]
      (junction 682) -> (junction 689) [order 2]
      (junction 687) -> (junction 691) : {lastClutchCom = clutchCom[0];
          |  Clutch_setValue(clutchCom[1]);}
    note: In caso di problema si riporta in endurance
    state checkShift [function]
      (default) -> (junction 635)
      (junction 635) -> (junction 637) [order 1] : [shiftCom[0] ~= lastShiftCom]
      (junction 635) -> (junction 641) [order 2]
      (junction 637) -> (junction 448) : {lastShiftCom = shiftCom[0];}
      (junction 448) -> (junction 450) [order 1] : [ shiftCom[1] == GEAR_COMMAND_UP]
      (junction 448) -> (junction 454) [order 2]
      (junction 450) -> (junction 452) : {send(GearshiftUp, NEUTRAL_STATE);
          |  send(GearshiftUp, GEARSHIFT);}
      (junction 454) -> (junction 456) [order 1] : [shiftCom[1] == GEAR_COMMAND_DOWN]
      (junction 454) -> (junction 460) [order 2]
      (junction 456) -> (junction 458) : {send(GearshiftDown, NEUTRAL_STATE);
          |  send(GearshiftDown, GEARSHIFT);}
      (junction 460) -> (junction 462) [order 1] : [shiftCom[1] == GEAR_COMMAND_NEUTRAL_UP]
      (junction 460) -> (junction 466) [order 2]
      (junction 462) -> (junction 464) : {send(GearshiftSetNeutral, NEUTRAL_STATE);
          |  send(GearshiftUp, GEARSHIFT);}
      (junction 466) -> (junction 469) [order 1] : [shiftCom[1] == GEAR_COMMAND_NEUTRAL_DOWN]
      (junction 466) -> (junction 473) [order 2]
      (junction 469) -> (junction 471) : {send(GearshiftSetNeutral, NEUTRAL_STATE);
          |  send(GearshiftDown, GEARSHIFT); }
    state ACCELERATION
      entry:
      lastModeCom[0] = modeCom[0];
      lastModeCom[1] = modeCom[1];
      state AAC
        note: Ricorda load dei default parameters
        note: Forse serve stato OFF, forse no
        note: ATTENZIONE: mancano delle istruzioni in alcuni stati
        note: E' giusto che clutch venga settata due volte?
        note: Riguarda funzionamento counter
        state ACTIVE
          note: Quindi continuo a settare Clutch?
          state START
            entry:
            accFb = 2;
            aacCounter = AAC_WORK_RATE_ms
            send(Efi_setRPMLimiter);
            Clutch_setValue(uint8(100));
            sendUpdatesSW(ACC_CODE, uint16(1));
            during:
            aacCounter = aacCounter - 1;
          state READY
            entry:
            accFb = 3;
            aacCounter = AAC_WORK_RATE_ms
            Clutch_setValue(uint8(100));
            during:
            aacCounter = aacCounter - 1;
            en, du:
            checkShift();
          note: SET blip è sbagliato
          state START_RELEASE
            entry:
            aac_clutchValue = double(getAacParam(RAMP_START));
            Clutch_setValue(uint8(aac_clutchValue));
            aac_dtRelease = getAacParam(RAMP_TIME) / int32(AAC_WORK_RATE_ms);
            aac_clutchStep = double((getAacParam(RAMP_START) - getAacParam(RAMP_END)) * int32(AAC_WORK_RATE_ms)) / double(getAacParam(RAMP_TIME));
            aacCounter = AAC_WORK_RATE_ms;
            sendUpdatesSW(ACC_CODE, uint16(2));
            during:
            aacCounter = aacCounter - 1;
          state RUNNING
            entry:
            aacCounter = AAC_WORK_RATE_ms
            lastShift =  currentGear;
            entry, during:
            aacCheckShift();
          note: Continuo a controllare ogni 25ms?
          state aacCheckShift [function]
            (default) -> (junction 716)
            (junction 716) -> (junction 717) [order 1] : [lastShift == currentGear]
            (junction 716) -> (junction 720) [order 2]
            (junction 717) -> (junction 593)
            (junction 593) -> (junction 604) [order 1] : [aac_externValues[int32(aac_values.RPM)] >= aac_parameters[ uint8(aac_params.RPM_LIMIT_1_2) + currentGear -1]]
            (junction 593) -> (junction 606) [order 2]
            (junction 604) -> (junction 608)
            (junction 608) -> (junction 610) [order 1] : [aac_externValues[int32(aac_values.WHEEL_SPEED)] >= aac_parameters[ uint8(aac_params.SPEED_LIMIT_1_2) + currentGear-1]]
            (junction 608) -> (junction 612) [order 2]
            (junction 610) -> (junction 614) : {send(GearshiftUp, GEARSHIFT); lastShift = lastShift + 1;}
          state RELEASING
            entry:
            aac_clutchValue = aac_clutchValue - aac_clutchStep;
            Clutch_setValue(uint8(aac_clutchValue));
            aac_dtRelease = aac_dtRelease - 1;
            aacCounter = AAC_WORK_RATE_ms;
            during:
            aacCounter = aacCounter - 1;
          note: Teniamo questa cosa di eseguire ogni 25ms? O calcoliamo direttamente
              | il Ttot?
          (default) -> MODES.ACCELERATION.AAC.ACTIVE.START
          (junction 558) -> READY [order 2]
          MODES.ACCELERATION.AAC.ACTIVE.START -> READY : [aacCounter <= 1]
          READY -> (junction 558) : [aacCounter <= 1]
          (junction 558) -> START_RELEASE [order 1] : [aacCom[0] ~= lastAacCom && aacCom[1] == RELEASE_AAC_COM]{lastAacCom = aacCom[0];}
          START_RELEASE -> RELEASING : [aacCounter <= 1]
          (junction 572) -> RUNNING [order 1] : [aac_dtRelease <= 0 || clutchCurrVal <= getAacParam(RAMP_END)]
              | {Clutch_setValue(uint8(0)); send(Efi_unsetRPMLimiter);}
          (junction 572) -> RELEASING [order 2]
          RELEASING -> (junction 572) : [aacCounter <=1]
        note: Quando devo fare clutch release?Forse risolto in CAN
        state STOPPING
          entry:
          send(Efi_unsetRPMLimiter);
          sendUpdatesSW(ACC_CODE, uint16(0));
        note: da verificare la marcia di uscita
        note: !!!!Gli array di MATLAB sono 1-based
        state param = getAacParam(index) [function]
          (default) -> (junction 566)
          (junction 566) -> (junction 570) : {param = aac_parameters[int32(index)]}
        ACTIVE -> STOPPING : [aacCom[0] ~= lastAacCom && aacCom[1] == STOP_AAC_COM]
            | {lastAacCom = aacCom[0]}
        RUNNING -> STOPPING : [currentGear == 5]
      state NotReady
        entry, during:
        accFb = 1;
        checkShift();
        checkClutch();
      note: prima di entrare svuotare il buffer
      (default) -> NotReady
      NotReady -> ACTIVE : [aacCom[0] ~= lastAacCom && aacCom[1] == START_AAC_COM]
          | {lastAacCom = aacCom[0]}
      STOPPING -> NotReady
    note: Stopping potrebbe essere esterno ad AAC,
        | Dove faccio unsetRPMLimiter?
    (junction 826) -> (junction 800)
    (default) -> MODES.INIT
    MODES.INIT -> (junction 800)
    (junction 800) -> AUTOCROSS [order 1] : [modeCom[1] == AUTOCROSS_MODE]
    (junction 800) -> (junction 808) [order 2]
    MANUAL_MODES -> (junction 826) : [modeCom[0] != lastModeCom[0] && modeCom[1] != lastModeCom[1]]
    ACCELERATION -> (junction 826) : [modeCom[0]~= lastModeCom[0] && modeCom[1] != lastModeCom[1]]
        | {send(Efi_unsetRPMLimiter)}
    (junction 808) -> ENDURANCE [order 1] : [modeCom[1] == ENDURANCE_MODE]
    (junction 808) -> (junction 812) [order 2]
    (junction 812) -> SKIDPAD [order 1] : [modeCom[1] == SKIDPAD_MODE]
    (junction 812) -> (junction 815) [order 2]
    (junction 815) -> MANUAL_MODES [order 2]
    (junction 815) -> ACCELERATION [order 1] : [modeCom[1] == ACC_MODE]
  note: DIVERSA DA QUELLA IN C E NON COMPLETA
  state sendUpdatesSW (valCode, value) [function]
  state NEUTRAL_STATE [parallel]
    settings: executionOrder=2
    state NEUTRAL
    state UNSET_NEUTRAL
    state SET_NEUTRAL
    state NO_NEUTRAL
    NEUTRAL -> UNSET_NEUTRAL [order 2] : GearshiftDown
    (default) -> NEUTRAL
    NEUTRAL -> UNSET_NEUTRAL [order 1] : GearshiftUp
    SET_NEUTRAL -> NEUTRAL : [in(GEARSHIFT.DOWN_END) || in(GEARSHIFT.UP_END)]
    UNSET_NEUTRAL -> NO_NEUTRAL : [in(GEARSHIFT.DOWN_END) || in(GEARSHIFT.UP_END)]
    NO_NEUTRAL -> SET_NEUTRAL : GearshiftSetNeutral
  state GEARSHIFT [parallel]
    settings: executionOrder=3
    state UPSHIFTING
      state UP_REBOUND
        entry:
        ticksCounter = Gearshift_getTime();
        during:
        ticksCounter = ticksCounter - 1;
        state Default
          entry:
          send(Gearshift_rebound);
        state SettingNeutral
          entry:
          Clutch_setValue(uint8(0));
          send(Gearshift_rebound);
        (default) -> (junction 392)
        (junction 392) -> GEARSHIFT.UPSHIFTING.UP_REBOUND.Default [order 2]
        (junction 392) -> GEARSHIFT.UPSHIFTING.UP_REBOUND.SettingNeutral [order 1] : [in(NEUTRAL_STATE.SET_NEUTRAL)]
      state UP_PUSH
        entry:
        ticksCounter = Gearshift_getTime();
        during:
        ticksCounter = ticksCounter - 1;
        state Default
          entry:
          send(Gearshift_up_push);
        state CutOff
          entry:
          send(Efi_unsetCut);
          send(Gearshift_up_push);
        (default) -> (junction 424)
        (junction 424) -> GEARSHIFT.UPSHIFTING.UP_PUSH.Default [order 2]
        (junction 424) -> CutOff [order 1] : [~in(NEUTRAL_STATE.SET_NEUTRAL)]
      state UP_START
        entry:
        ticksCounter = Gearshift_getTime();
        during:
        ticksCounter = ticksCounter - 1;
        state Default
          entry:
          Efi_setCut;
        state SettingNeutral
          entry:
          Clutch_setValue(uint8(80));
        (default) -> (junction 386)
        (junction 386) -> GEARSHIFT.UPSHIFTING.UP_START.Default [order 2]
        (junction 386) -> GEARSHIFT.UPSHIFTING.UP_START.SettingNeutral [order 1] : [in(NEUTRAL_STATE.SET_NEUTRAL)]
      state UP_BRAKE
        entry:
        ticksCounter = Gearshift_getTime();
        send(Gearshift_brake);
        during:
        ticksCounter = ticksCounter - 1;
      UP_REBOUND -> UP_BRAKE : [ticksCounter == 0]
      UP_START -> UP_PUSH : [ticksCounter == 0]
      UP_PUSH -> UP_REBOUND : [ticksCounter == 0]
    state UP_END
      entry:
      send(Gearshift_free);
    state IDLE
    state INIT
      entry:
      ticksCounter = 0;
    note: Ricorda inizializzare CLUTCH
    state DOWNSHIFTING
      state DOWN_START
        entry:
        ticksCounter = Gearshift_getTime();
        during:
        ticksCounter = ticksCounter - 1;
        state SettingNeutral
          entry:
          Clutch_setValue(uint8(80));
        state ChangeClutch
          entry:
          Clutch_setValue(uint8(60));
        state Default
        (default) -> (junction 400)
        (junction 400) -> GEARSHIFT.DOWNSHIFTING.DOWN_START.SettingNeutral [order 1] : [in(NEUTRAL_STATE.SET_NEUTRAL)  &&  clutchCurrVal <= 80]
        (junction 400) -> (junction 403) [order 2]
        (junction 403) -> GEARSHIFT.DOWNSHIFTING.DOWN_START.ChangeClutch [order 1] : [~in(NEUTRAL_STATE.UNSET_NEUTRAL) && clutchCurrVal <= 60]
        (junction 403) -> GEARSHIFT.DOWNSHIFTING.DOWN_START.Default [order 2]
      state DOWN_BRAKE
        entry:
        ticksCounter =Gearshift_getTime();
        during:
        ticksCounter = ticksCounter - 1;
        state Default
          entry:
          send(Gearshift_brake);
        state ChangeClutch
          entry:
          Clutch_setValue(uint8(80));
          send(Gearshift_brake);
        (default) -> (junction 411)
        (junction 411) -> GEARSHIFT.DOWNSHIFTING.DOWN_BRAKE.Default [order 2]
        (junction 411) -> GEARSHIFT.DOWNSHIFTING.DOWN_BRAKE.ChangeClutch [order 1] : [clutchCurrVal < 81]
      state DOWN_PUSH
        entry:
        ticksCounter = Gearshift_getTime();
        send(Gearshift_down_push);
        during:
        ticksCounter = ticksCounter - 1;
      state DOWN_REBOUND
        entry:
        ticksCounter = Gearshift_getTime();
        send(Gearshift_rebound);
        during:
        ticksCounter = ticksCounter - 1;
      DOWN_START -> DOWN_PUSH : [ticksCounter == 0]
      DOWN_REBOUND -> DOWN_BRAKE : [ticksCounter == 0]
      DOWN_PUSH -> DOWN_REBOUND : [ticksCounter == 0]
    state DOWN_END
      entry:
      send(Gearshift_free);
    state time = Gearshift_getTime [function]
      (default) -> (junction 238)
      (junction 238) -> (junction 240) [order 1] : [in(UPSHIFTING.UP_START)]
      (junction 240) -> (junction 271) [order 1] : [in(NEUTRAL_STATE.SET_NEUTRAL)]
      (junction 238) -> (junction 241) [order 2]
      (junction 240) -> (junction 322) [order 2] : {time = int32(timings.DEFAULT_DELAY);}
      (junction 271) -> (junction 275) : {time = int32(timings.DEFAULT_NT_CLUTCH_DELAY);}
      (junction 347) -> (junction 348) [order 1] : [in(NEUTRAL_STATE.SET_NEUTRAL)]
      (junction 241) -> (junction 347) [order 1] : [in(UPSHIFTING.UP_PUSH)]
      (junction 347) -> (junction 359) [order 2]
      (junction 348) -> (junction 363) : {time = int32(timings.DEFAULT_NT_CLUTCH_DELAY)}
      (junction 241) -> (junction 243) [order 2]
      (junction 244) -> (junction 324) [order 1] : [in(NEUTRAL_STATE.SET_NEUTRAL)]
      (junction 243) -> (junction 244) [order 1] : [in(UPSHIFTING.UP_REBOUND)]
      (junction 243) -> (junction 245) [order 2]
      (junction 244) -> (junction 326) [order 2] : {time = int32(timings.DEFAULT_UP_REBOUND);}
      (junction 324) -> (junction 327) : {time = int32(timings.DEFAULT_NT_REBOUND_1_N);}
      (junction 359) -> (junction 360) [order 1] : [currentGear == 1]
      (junction 360) -> (junction 365) : {time = int32(timings.DEFAULT_UP_PUSH_1_2)}
      (junction 359) -> (junction 351) [order 2]
      (junction 245) -> (junction 246) [order 1] : [in(UPSHIFTING.UP_BRAKE)]
      (junction 246) -> (junction 330) [order 1] : [in(NEUTRAL_STATE.SET_NEUTRAL)]
      (junction 351) -> (junction 362) [order 1] : [currentGear == 2]
      (junction 362) -> (junction 367) : {time = int32(timings.DEFAULT_UP_PUSH_2_3)}
      (junction 245) -> (junction 247) [order 2]
      (junction 246) -> (junction 332) [order 2] : {time = int32(timings.DEFAULT_UP_BRAKE);}
      (junction 330) -> (junction 333) : {time = int32(timings.DEFAULT_NT_BRAKE_1_N);}
      (junction 351) -> (junction 355) [order 2]
      (junction 247) -> (junction 248) [order 1] : [in(DOWNSHIFTING.DOWN_START)]
      (junction 355) -> (junction 344) [order 1] : [currentGear == 3]
      (junction 344) -> (junction 369) : {time = int32(timings.DEFAULT_UP_PUSH_3_4)}
      (junction 247) -> (junction 249) [order 2]
      (junction 248) -> (junction 336) : {time = int32(timings.DEFAULT_CLUTCH);}
      (junction 355) -> (junction 356) [order 2]
      (junction 249) -> (junction 250) [order 1] : [in(DOWNSHIFTING.DOWN_PUSH)]
      (junction 356) -> (junction 354) [order 1] : [currentGear == 4]
      (junction 354) -> (junction 371) : {time = int32(timings.DEFAULT_UP_PUSH_4_5)}
      (junction 249) -> (junction 251) [order 2]
      (junction 250) -> (junction 338) : {time = int32(timings.DEFAULT_DN_PUSH);}
      (junction 356) -> (junction 342) [order 2] : {time = int32(timings.DEFAULT_UP_PUSH_2_3)}
      (junction 251) -> (junction 252) [order 1] : [in(DOWNSHIFTING.DOWN_REBOUND)]
      (junction 251) -> (junction 254) [order 2] : {time = int32(timings.DEFAULT_DN_BRAKE);}
      (junction 252) -> (junction 340) : {time = int32(timings.DEFAULT_DN_REBOUND);}
    UP_BRAKE -> UP_END : [ticksCounter == 0]
    IDLE -> UP_START [order 1] : GearshiftUp
    UP_END -> IDLE
    (default) -> GEARSHIFT.INIT
    GEARSHIFT.INIT -> IDLE
    DOWN_END -> IDLE
    IDLE -> DOWN_START [order 2] : GearshiftDown
    DOWN_BRAKE -> DOWN_END : [ticksCounter == 0]
  state Clutch_setValue(setValue) [function]
    (default) -> (junction 503)
    (junction 503) -> (junction 504) : {clutchCurrVal = setValue; send(Clutch_set);}
  note: Verifica che il controllo su min/max non sia necessario
  state START_ENGINE [parallel]
    settings: executionOrder=4
    state WAIT
    state START
      entry:
      send(EngineControl_start);
      lastCom = startEngCom;
      startCounter = 100;
      during:
      startCounter = startCounter - 1;
    state STOP
      entry:
      send(EngineControl_stop);
    (default) -> WAIT
    WAIT -> (junction 496)
    START_ENGINE.START -> (junction 496) [order 2] : [startEngCom != lastCom]
    (junction 496) -> START_ENGINE.START : [startEngCom != lastCom]
    STOP -> (junction 496)
    START_ENGINE.START -> STOP [order 1] : [startCounter <= 0]
  state SENSORS [parallel]
    settings: executionOrder=5
  data: GEAR_COMMAND_NEUTRAL_UP constant uint16 =uint16(50); GEAR_COMMAND_NEUTRAL_DOWN constant uint16 =uint16(100); GEAR_COMMAND_UP constant uint16 =uint16(400); GEAR_COMMAND_DOWN constant uint16 =uint16(200); GEAR_COMMAND_NEUTRAL_UP constant uint16 =uint16(50); GEAR_COMMAND_NEUTRAL_DOWN constant uint16 =uint16(100); GEAR_COMMAND_UP constant uint16 =uint16(400); GEAR_COMMAND_DOWN constant uint16 =uint16(200); index function_input Enum: aac_params size=1; param function_output int32 size=1; aac_parameters local int32 size=[1,11] =aacParameters; AAC_WORK_RATE_ms constant uint16 =uint16(25); aacCounter local uint16 size=1; aac_clutchValue local double size=1 =0; aac_clutchStep local double size=1; aac_dtRelease local int32 size=1; DEF_RAMP_START constant int32 =int32(50); DEF_RAMP_END constant int32 =int32(0); DEF_RAMP_TIME constant int32 =int32(250); DEF_RPM_LIMIT_1_2 constant int32 =int32(11000); DEF_RPM_LIMIT_2_3 constant int32 =int32(11000); DEF_RPM_LIMIT_3_4 constant int32 =int32(11000); DEF_RPM_LIMIT_4_5 constant int32 =int32(11000); DEF_SPEED_LIMIT_1_2 constant int32 =int32(46); DEF_SPEED_LIMIT_2_3 constant int32 =int32(61); DEF_SPEED_LIMIT_3_4 constant int32 =int32(77); DEF_SPEED_LIMIT_4_5 constant int32 =int32(113); ACC_CODE constant uint16 =uint16(1); lastAacCom local uint16 size=1 =uint16(0); START_AAC_COM constant uint16 =uint16(1); RELEASE_AAC_COM constant uint16 =uint16(2); STOP_AAC_COM constant uint16 =uint16(0); lastShiftCom local uint16 size=1 =uint16(0); lastClutchCom local uint8 size=1 =uint8(0); AUTOCROSS_MODE constant uint16 =uint16(0); SKIDPAD_MODE constant uint16 =uint16(1); ENDURANCE_MODE constant uint16 =uint16(2); ACC_MODE constant uint16 =uint16(3); valCode function_input uint16 size=1; value function_input uint16 size=1; time function_output int32 size=1; ticksCounter local int32 size=1; data constant double; setValue function_input uint8 size=1; lastCom local uint8 size=1 =uint8(0); startCounter local uint8 size=1; currentGear input uint8 size=1 =0; clutchCurrVal output uint8 size=1 [uint8(0)..uint8(100)] =uint8(0); lastModeCom output uint16 size=2 =uint16(0); shiftCom input uint16 size=[1,2]; startEngCom input uint8 size=1; aacCom input uint16 size=[1,2]; aac_externValues input uint16 size=[1,3]; clutchCom input uint8 size=[1,2]; lastShift local uint8 size=1 =uint8(0);; modeCom input uint16 size=[1,2]; accFb output uint16 =uint16(0)
  events: Clutch_init output FUNCTION_CALL_EVENT; Clutch_set output FUNCTION_CALL_EVENT; Efi_init output FUNCTION_CALL_EVENT; Efi_setCut output FUNCTION_CALL_EVENT; Efi_unsetCut output FUNCTION_CALL_EVENT; Efi_setRPMLimiter output FUNCTION_CALL_EVENT; Efi_unsetRPMLimiter output FUNCTION_CALL_EVENT; Gearshift_rebound output FUNCTION_CALL_EVENT; Gearshift_up_push output FUNCTION_CALL_EVENT; Gearshift_down_push output FUNCTION_CALL_EVENT; Gearshift_brake output FUNCTION_CALL_EVENT; Gearshift_free output FUNCTION_CALL_EVENT; GearshiftUp local FUNCTION_CALL_EVENT; GearshiftDown local FUNCTION_CALL_EVENT; GearshiftSetNeutral local FUNCTION_CALL_EVENT; EngineControl_start output FUNCTION_CALL_EVENT; EngineControl_stop output FUNCTION_CALL_EVENT
